simulink model "Headlamp_Leveling_System_Sim"  (R2019b)
settings: Solver=VariableStepAuto  StartTime=0.0  StopTime=1.0  RelTol=1e-3
libraries: simulink x2
settings Model: Creator=Bogdan  LastModifiedBy=Bogdan
settings DebuggingCC: AlgebraicLoopMsg=none

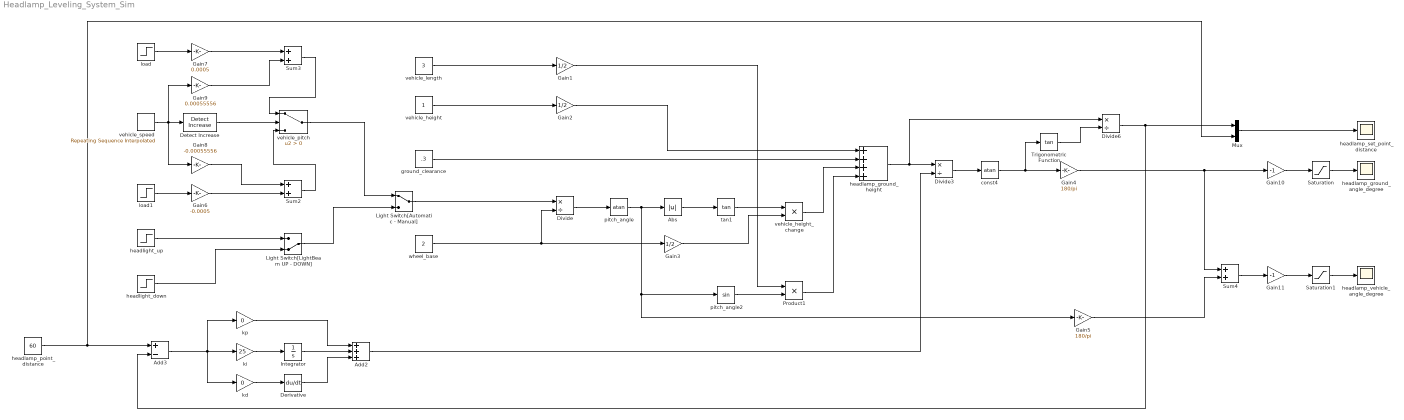
== system Headlamp_Leveling_System_Sim ==
  Abs : Abs
  Add2 : Sum  Inputs=+++
  Add3 : Sum  Inputs=+-
  Derivative : Derivative
  Detect Increase : simulink/Logic and Bit Operations/Detect Increase  vinit=0.0  OutDataTypeStr=uint8
  Divide : Product  Inputs=*/
  Divide3 : Product  Inputs=*/  RndMeth=Ceiling
  Divide6 : Product  Inputs=*/
  Gain1 : Gain  Gain=1/2
  Gain10 : Gain  Gain=-1
  Gain11 : Gain  Gain=-1
  Gain2 : Gain  Gain=1/2
  Gain3 : Gain  Gain=1/2
  Gain4 : Gain  Gain=180/pi
  Gain5 : Gain  Gain=180/pi
  Gain6 : Gain  Gain=-0.0005
  Gain7 : Gain  Gain=0.0005
  Gain8 : Gain  Gain=-0.00055556
  Gain9 : Gain  Gain=0.00055556
  Integrator : Integrator
  Light Switch[Automatic - Manual] : ManualSwitch
  Light Switch[LightBeam UP - DOWN] : ManualSwitch  CurrentSetting=0
  Mux : Mux  Inputs=2
  Product1 : Product
  Saturation : Saturate  UpperLimit=2  LowerLimit=-2
  Saturation1 : Saturate  UpperLimit=20  LowerLimit=-20
  Sum2 : Sum
  Sum3 : Sum
  Sum4 : Sum
  Trigonometric Function : Trigonometry  Operator=tan
  const4 : Trigonometry  Operator=atan
  ground_clearance : Constant  Value=.3
  headlamp_ground_angle_degree : Scope
  headlamp_ground_height : Sum  Inputs=++++
  headlamp_point_distance : Constant  Value=60
  headlamp_set_point_distance : Scope
  headlamp_vehicle_angle_degree : Scope
  headlight_down : Step  Time=.4  After=-0.2  SampleTime=0
  headlight_up : Step  Time=.4  After=0.2  SampleTime=0
  kd : Gain  Gain=0
  ki : Gain  Gain=25
  kp : Gain  Gain=0
  load : Step  Time=0  After=300  SampleTime=0
  load1 : Step  Time=0  After=300  SampleTime=0
  pitch_angle : Trigonometry  Operator=atan
  pitch_angle2 : Trigonometry
  tan1 : Trigonometry  Operator=tan
  vehicle_height : Constant
  vehicle_height_change : Product
  vehicle_length : Constant  Value=3
  vehicle_pitch : Switch  Criteria=u2 > Threshold
  vehicle_speed : simulink/Sources/Repeating Sequence Interpolated  OutValues=[60 10 90 120 0].'  TimeValues=[0 .2 .4 .6 1].'  LookUpMeth=Interpolation-Use End Values  tsamp=0.001  OutMin=[]  OutMax=[]  OutDataTypeStr=double  OutputDataTypeScalingMode=double  OutDataType=fixdt(0,8)  OutScaling=2^-10
  wheel_base : Constant  Value=2
  wires:
  wheel_base/1 -> Divide/2, Gain3/1
  Sum4/1 -> Gain11/1
  vehicle_height/1 -> Gain2/1
  Divide6/1 -> Add3/2, Mux/1
  Add3/1 -> kp/1, kd/1, ki/1
  headlamp_point_distance/1 -> Add3/1, Mux/2
  headlamp_ground_height/1 -> Divide3/1, Divide6/1
  Gain1/1 -> Product1/1
  Trigonometric Function/1 -> Divide6/2
  ki/1 -> Integrator/1
  Gain5/1 -> Sum4/2
  Derivative/1 -> Add2/3
  Add2/1 -> Divide3/2
  tan1/1 -> vehicle_height_change/1
  vehicle_length/1 -> Gain1/1
  Mux/1 -> headlamp_set_point_distance/1
  kd/1 -> Derivative/1
  kp/1 -> Add2/1
  pitch_angle/1 -> Gain5/1, pitch_angle2/1, Abs/1
  Abs/1 -> tan1/1
  Divide/1 -> pitch_angle/1
  Gain4/1 -> Sum4/1, Gain10/1
  Gain2/1 -> headlamp_ground_height/1
  pitch_angle2/1 -> Product1/2
  Divide3/1 -> const4/1
  ground_clearance/1 -> headlamp_ground_height/2
  Product1/1 -> headlamp_ground_height/4
  Integrator/1 -> Add2/2
  Gain3/1 -> vehicle_height_change/2
  const4/1 -> Trigonometric Function/1, Gain4/1
  vehicle_height_change/1 -> headlamp_ground_height/3
  Detect Increase/1 -> vehicle_pitch/2
  load1/1 -> Gain6/1
  Gain6/1 -> Sum2/2
  Light Switch[Automatic - Manual]/1 -> Divide/1
  Gain8/1 -> Sum2/1
  vehicle_speed/1 -> Gain9/1, Gain8/1, Detect Increase/1
  Gain7/1 -> Sum3/1
  Gain9/1 -> Sum3/2
  load/1 -> Gain7/1
  Sum3/1 -> vehicle_pitch/1
  Sum2/1 -> vehicle_pitch/3
  Saturation/1 -> headlamp_ground_angle_degree/1
  Saturation1/1 -> headlamp_vehicle_angle_degree/1
  headlight_up/1 -> Light Switch[LightBeam UP - DOWN]/1
  headlight_down/1 -> Light Switch[LightBeam UP - DOWN]/2
  vehicle_pitch/1 -> Light Switch[Automatic - Manual]/1
  Light Switch[LightBeam UP - DOWN]/1 -> Light Switch[Automatic - Manual]/2
  Gain10/1 -> Saturation/1
  Gain11/1 -> Saturation1/1
